simulink model "IEEE_9bus"  (R2018b)
settings: Solver=VariableStepAuto  StartTime=0.0  StopTime=10.0  FixedStep=0.0001  RelTol=1e-3
values from neighbouring files (symbols this model uses):
  R12 = 0.0180    (= 0.018)    [IEEE9BUSdata.m]
  R14 = 0.015    [IEEE9BUSdata.m]
  R23 = 0.018    [IEEE9BUSdata.m]
  R39 = 0.02    [IEEE9BUSdata.m]
  R45 = 0.013    [IEEE9BUSdata.m]
  R46 = 0.02    [IEEE9BUSdata.m]
  R57 = 0.014    [IEEE9BUSdata.m]
  R69 = 0.01    [IEEE9BUSdata.m]
  R78 = 0.032    [IEEE9BUSdata.m]
  R89 = 0.022    [IEEE9BUSdata.m]
  Xc12 = 0.0045    [IEEE9BUSdata.m]
  Xc14 = 0.0038    [IEEE9BUSdata.m]
  Xc23 = 0.00    (= 0)    [IEEE9BUSdata.m]
  Xc39 = 0.00    (= 0)    [IEEE9BUSdata.m]
  Xc45 = 0.003    [IEEE9BUSdata.m]
  Xc46 = 0.00    (= 0)    [IEEE9BUSdata.m]
  Xc57 = 0.003    [IEEE9BUSdata.m]
  Xc69 = 0.00    (= 0)    [IEEE9BUSdata.m]
  Xc78 = 0.00    (= 0)    [IEEE9BUSdata.m]
  Xc89 = 0.00    (= 0)    [IEEE9BUSdata.m]
  Xl12 = 0.054    [IEEE9BUSdata.m]
  Xl14 = 0.045    [IEEE9BUSdata.m]
  Xl23 = 0.056    [IEEE9BUSdata.m]
  Xl39 = 0.06    [IEEE9BUSdata.m]
  Xl45 = 0.036    [IEEE9BUSdata.m]
  Xl46 = 0.066    [IEEE9BUSdata.m]
  Xl57 = 0.036    [IEEE9BUSdata.m]
  Xl69 = 0.05    [IEEE9BUSdata.m]
  Xl78 = 0.076    [IEEE9BUSdata.m]
  Xl89 = 0.065    [IEEE9BUSdata.m]
libraries: powerlib x32
settings Model: Creator=033-18-0019  LastModifiedBy=033-18-0019

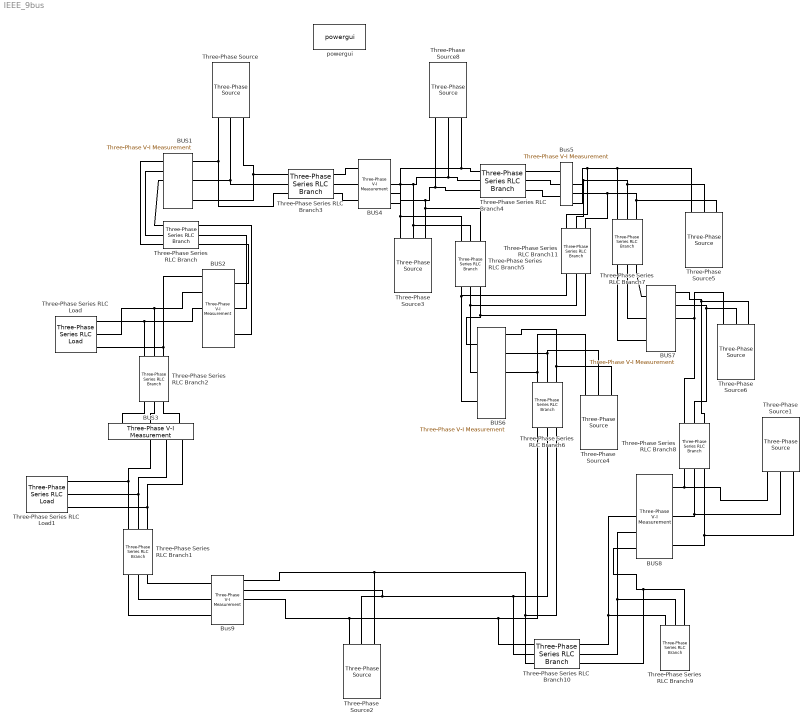
== system IEEE_9bus ==
  BUS1 : powerlib/Measurements/Three-Phase V-I Measurement  VoltageMeasurement=phase-to-ground  SetLabelV=off  LabelV=Vb1  Vpu=off  VpuLL=off  CurrentMeasurement=yes  SetLabelI=off  LabelI=Ib1  Ipu=off  Pbase=100e6  Vbase=500e3  OutputType=Complex  PhasorSimulation=off  PSBequivalent=0  mask(Three-Phase VI Measurement){}
      mask Display:
      | % This is a new mask on top of the base mask.
      | % Use "View base mask" link below to see the base mask.
      | disp('Bus1')
  BUS2 : powerlib/Measurements/Three-Phase V-I Measurement  VoltageMeasurement=phase-to-ground  SetLabelV=off  LabelV=Vabc  Vpu=off  VpuLL=off  CurrentMeasurement=yes  SetLabelI=off  LabelI=Iabc  Ipu=off  Pbase=100e6  Vbase=500e3  OutputType=Complex  PhasorSimulation=off  PSBequivalent=0  mask(Three-Phase VI Measurement){}
      mask Display:
      | % This is a new mask on top of the base mask.
      | % Use "View base mask" link below to see the base mask.
      | disp('Bus2')
  "BUS3 " : powerlib/Measurements/Three-Phase V-I Measurement  VoltageMeasurement=phase-to-ground  SetLabelV=off  LabelV=Vabc  Vpu=off  VpuLL=off  CurrentMeasurement=yes  SetLabelI=off  LabelI=Iabc  Ipu=off  Pbase=100e6  Vbase=500e3  OutputType=Complex  PhasorSimulation=off  PSBequivalent=0  mask(Three-Phase VI Measurement){}
      mask Display:
      | % This is a new mask on top of the base mask.
      | % Use "View base mask" link below to see the base mask.
      | disp('Bus3')
  BUS4 : powerlib/Measurements/Three-Phase V-I Measurement  VoltageMeasurement=phase-to-ground  SetLabelV=off  LabelV=Vb4  Vpu=on  VpuLL=off  CurrentMeasurement=yes  SetLabelI=off  LabelI=Ib4  Ipu=off  Pbase=100e6  Vbase=500e3  OutputType=Complex  PhasorSimulation=off  PSBequivalent=0
  BUS6 : powerlib/Measurements/Three-Phase V-I Measurement  VoltageMeasurement=phase-to-ground  SetLabelV=off  LabelV=Vb6  Vpu=on  VpuLL=off  CurrentMeasurement=yes  SetLabelI=off  LabelI=Ib6  Ipu=off  Pbase=100e6  Vbase=500e3  OutputType=Complex  PhasorSimulation=off  PSBequivalent=0
  BUS7 : powerlib/Measurements/Three-Phase V-I Measurement  VoltageMeasurement=phase-to-ground  SetLabelV=off  LabelV=Vb7  Vpu=on  VpuLL=off  CurrentMeasurement=yes  SetLabelI=off  LabelI=Ib7  Ipu=off  Pbase=100e6  Vbase=500e3  OutputType=Complex  PhasorSimulation=off  PSBequivalent=0
  BUS8 : powerlib/Measurements/Three-Phase V-I Measurement  VoltageMeasurement=phase-to-ground  SetLabelV=off  LabelV=Vb8  Vpu=off  VpuLL=off  CurrentMeasurement=yes  SetLabelI=off  LabelI=Ib8  Ipu=off  Pbase=100e6  Vbase=500e3  OutputType=Complex  PhasorSimulation=off  PSBequivalent=0
  Bus5 : powerlib/Measurements/Three-Phase V-I Measurement  VoltageMeasurement=phase-to-ground  SetLabelV=off  LabelV=V5  Vpu=on  VpuLL=off  CurrentMeasurement=yes  SetLabelI=off  LabelI=I5  Ipu=off  Pbase=100e6  Vbase=500e3  OutputType=Complex  PhasorSimulation=off  PSBequivalent=0
  Bus9 : powerlib/Measurements/Three-Phase V-I Measurement  VoltageMeasurement=phase-to-ground  SetLabelV=off  LabelV=Vb9  Vpu=on  VpuLL=off  CurrentMeasurement=yes  SetLabelI=off  LabelI=Ib9  Ipu=off  Pbase=100e6  Vbase=500e3  OutputType=Complex  PhasorSimulation=off  PSBequivalent=0
  Three-Phase Series RLC Branch : powerlib/Elements/Three-Phase Series RLC Branch  LConnTagsString=A|B|C  RConnTagsString=A|B|C  BranchType=RLC  Resistance=R12  Inductance=2*pi*50*Xl12  Capacitance=1/(2*pi*50*Xc12)  Measurements=None
  Three-Phase Series RLC Branch1 : powerlib/Elements/Three-Phase Series RLC Branch  LConnTagsString=A|B|C  RConnTagsString=A|B|C  BranchType=RLC  Resistance=R39  Inductance=2*pi*50*Xl39  Capacitance=1/(2*pi*50*Xc39)  Measurements=None
  Three-Phase Series RLC Branch10 : powerlib/Elements/Three-Phase Series RLC Branch  LConnTagsString=A|B|C  RConnTagsString=A|B|C  BranchType=RLC  Resistance=R89  Inductance=2*pi*50*Xl89  Capacitance=1/(2*pi*50*Xc89)  Measurements=None
  Three-Phase Series RLC Branch11 : powerlib/Elements/Three-Phase Series RLC Branch  LConnTagsString=A|B|C  RConnTagsString=A|B|C  BranchType=RLC  Resistance=R78  Inductance=2*pi*50*Xl78  Capacitance=1/(2*pi*50*Xc78)  Measurements=None
  Three-Phase Series RLC Branch2 : powerlib/Elements/Three-Phase Series RLC Branch  LConnTagsString=A|B|C  RConnTagsString=A|B|C  BranchType=RLC  Resistance=R23  Inductance=2*pi*50*Xl23  Capacitance=1/(2*pi*50*Xc23)  Measurements=None
  Three-Phase Series RLC Branch3 : powerlib/Elements/Three-Phase Series RLC Branch  LConnTagsString=A|B|C  RConnTagsString=A|B|C  BranchType=RLC  Resistance=R14  Inductance=2*pi*50*Xl14  Capacitance=1/(2*pi*50*Xc14)  Measurements=None
  Three-Phase Series RLC Branch4 : powerlib/Elements/Three-Phase Series RLC Branch  LConnTagsString=A|B|C  RConnTagsString=A|B|C  BranchType=RLC  Resistance=R45  Inductance=2*pi*50*Xl45  Capacitance=1/(2*pi*50*Xc45)  Measurements=None
  Three-Phase Series RLC Branch5 : powerlib/Elements/Three-Phase Series RLC Branch  LConnTagsString=A|B|C  RConnTagsString=A|B|C  BranchType=RLC  Resistance=R46  Inductance=2*pi*50*Xl46  Capacitance=1/(2*pi*50*Xc46)  Measurements=None
  Three-Phase Series RLC Branch6 : powerlib/Elements/Three-Phase Series RLC Branch  LConnTagsString=A|B|C  RConnTagsString=A|B|C  BranchType=RLC  Resistance=R69  Inductance=2*pi*50*Xl69  Capacitance=1/(2*pi*50*Xc69)  Measurements=None
  Three-Phase Series RLC Branch7 : powerlib/Elements/Three-Phase Series RLC Branch  LConnTagsString=A|B|C  RConnTagsString=A|B|C  BranchType=RLC  Resistance=R57  Inductance=2*pi*50*Xl57  Capacitance=1/(2*pi*50*Xc57)  Measurements=None
  Three-Phase Series RLC Branch8 : powerlib/Elements/Three-Phase Series RLC Branch  LConnTagsString=A|B|C  RConnTagsString=A|B|C  BranchType=RLC  Resistance=R78  Inductance=2*pi*50*Xl78  Capacitance=1/(2*pi*50*Xc78)  Measurements=None
  Three-Phase Series RLC Branch9 : powerlib/Elements/Three-Phase Series RLC Branch  LConnTagsString=A|B|C  RConnTagsString=A|B|C  BranchType=RLC  Resistance=R78  Inductance=2*pi*50*Xl78  Capacitance=1/(2*pi*50*Xc78)  Measurements=None
  Three-Phase Series RLC Load : powerlib/Elements/Three-Phase Series RLC Load  LConnTagsString=A|B|C  Configuration=Y (grounded)  NominalVoltage=1000  Vabc=[1e3 1e3 1e3]  Vabcp=[1e3 1e3 1e3]  NominalFrequency=60  UnbalancedPower=off  ActivePower=10e3  InductivePower=100  CapacitivePower=100  Pabc=[10e3 9e3 11e3]  QLabc=[100 90 110]  QCabc=[100 90 110]  Pabcp=[10e3 9e3 11e3]  QLabcp=[100 90 110]  QCabcp=[100 90 110]  Measurements=None  LoadType=constant Z
  Three-Phase Series RLC Load1 : powerlib/Elements/Three-Phase Series RLC Load  LConnTagsString=A|B|C  Configuration=Y (grounded)  NominalVoltage=1000  Vabc=[1e3 1e3 1e3]  Vabcp=[1e3 1e3 1e3]  NominalFrequency=60  UnbalancedPower=off  ActivePower=10e3  InductivePower=100  CapacitivePower=100  Pabc=[10e3 9e3 11e3]  QLabc=[100 90 110]  QCabc=[100 90 110]  Pabcp=[10e3 9e3 11e3]  QLabcp=[100 90 110]  QCabcp=[100 90 110]  Measurements=None  LoadType=constant Z
  Three-Phase Source : powerlib/Electrical Sources/Three-Phase Source  InternalConnection=Yg  VoltagePhases=off  Voltage=132e3  PhaseAngle=0  Voltage_phases=[25e3 25e3 25e3]/sqrt(3)  PhaseAngles_phases=[0 -120 +120]  Frequency=50  NonIdealSource=on  SpecifyImpedance=off  Resistance=0.8929  Inductance=0.05/(2*pi*50)  ShortCircuitLevel=100e6  BaseVoltage=132e3  XRratio=7  BusType=swing  Pref=10e3  Qref=0  Prefabc=[10e3, 10e3, 10e3]  Qrefabc=[0, 0, 0]  Qmin=-inf  Qmax=inf
  Three-Phase Source1 : powerlib/Electrical Sources/Three-Phase Source  InternalConnection=Yg  VoltagePhases=off  Voltage=132e3  PhaseAngle=0  Voltage_phases=[25e3 25e3 25e3]/sqrt(3)  PhaseAngles_phases=[0 -120 +120]  Frequency=50  NonIdealSource=on  SpecifyImpedance=off  Resistance=0.8929  Inductance=0.1/(2*pi*50)  ShortCircuitLevel=100e6  BaseVoltage=132e3  XRratio=7  BusType=swing  Pref=10e3  Qref=0  Prefabc=[10e3, 10e3, 10e3]  Qrefabc=[0, 0, 0]  Qmin=-inf  Qmax=inf
  Three-Phase Source{2..6} (5 alike) : powerlib/Electrical Sources/Three-Phase Source  InternalConnection=Yg  VoltagePhases=off  Voltage=25e3  PhaseAngle=0  Voltage_phases=[25e3 25e3 25e3]/sqrt(3)  PhaseAngles_phases=[0 -120 +120]  Frequency=60  NonIdealSource=on  SpecifyImpedance=off  Resistance=0.8929  Inductance=16.58e-3  ShortCircuitLevel=100e6  BaseVoltage=25e3  XRratio=7  BusType=swing  Pref=10e3  Qref=0  Prefabc=[10e3, 10e3, 10e3]  Qrefabc=[0, 0, 0]  Qmin=-inf  Qmax=inf
  Three-Phase Source8 : powerlib/Electrical Sources/Three-Phase Source  InternalConnection=Yg  VoltagePhases=off  Voltage=132e3  PhaseAngle=0  Voltage_phases=[25e3 25e3 25e3]/sqrt(3)  PhaseAngles_phases=[0 -120 +120]  Frequency=50  NonIdealSource=on  SpecifyImpedance=off  Resistance=0.8929  Inductance=0.08/(2*pi*50)  ShortCircuitLevel=100e6  BaseVoltage=132e3  XRratio=7  BusType=swing  Pref=10e3  Qref=0  Prefabc=[10e3, 10e3, 10e3]  Qrefabc=[0, 0, 0]  Qmin=-inf  Qmax=inf
  powergui : powerlib/powergui  Priority=1  SimulationMode=Discrete  SampleTime=50e-6  frequency=60  Iterations=50  frequencyindice=60  Pbase=100e6  ErrMax=1e-4  UnitsV=kV  UnitsW=MW  buscounter=0  FunctionMessages=off  echomessages=off  EnableUseOfTLC=off  CurrentSourceSwitches=off  DisableSnubberDevices=off  DisableRonSwitches=off  DisableVfSwitches=off  DisplayEquations=off  SolverType=Tustin/Backward Euler (TBE)  Interpol=off  ExternalGateDelay=off  methode=off  Ts=100  x0status=blocks  SPID=off  SwTol=0  HookPort=off  RestoreLinks=warning  ResistiveCurrentMeasurement=off  Frange=[0:2:500]  Ylog=off  Xlog=on  ShowGrid=off  save=off  variable=ZData  structure=0  ZoomFFT=off  StartTime=0.0  cycles=1  DisplayStyle=1  fundamental=60  FreqAxis=off  MaxFrequency=1000  frequencyindicesteady=1  RmsSteady=1  display=off
  connections:
  BUS4/LConn3 -- Three-Phase Series RLC Branch3/RConn3
  BUS4/LConn2 -- Three-Phase Series RLC Branch3/RConn2
  Three-Phase Source/RConn1 -- Three-Phase Series RLC Branch3/LConn1 -- BUS1/LConn1
  Three-Phase Series RLC Branch/RConn1 -- BUS2/LConn1
  Three-Phase Series RLC Branch/RConn2 -- BUS2/LConn2
  Three-Phase Series RLC Branch/RConn3 -- BUS2/LConn3
  Three-Phase Series RLC Branch/LConn1 -- BUS1/RConn1
  BUS1/RConn2 -- Three-Phase Series RLC Branch/LConn2
  BUS1/RConn3 -- Three-Phase Series RLC Branch/LConn3
  Three-Phase Series RLC Branch2/RConn1 -- "BUS3 "/LConn1
  "BUS3 "/LConn2 -- Three-Phase Series RLC Branch2/RConn2
  Three-Phase Series RLC Load/LConn3 -- BUS2/RConn3 -- Three-Phase Series RLC Branch2/LConn3
  "BUS3 "/RConn1 -- Three-Phase Series RLC Branch1/LConn1 -- Three-Phase Series RLC Load1/LConn1
  Three-Phase Series RLC Load1/LConn2 -- "BUS3 "/RConn2 -- Three-Phase Series RLC Branch1/LConn2
  "BUS3 "/RConn3 -- Three-Phase Series RLC Load1/LConn3 -- Three-Phase Series RLC Branch1/LConn3
  Three-Phase Series RLC Branch1/RConn1 -- Bus9/LConn1
  Three-Phase Series RLC Branch1/RConn2 -- Bus9/LConn2
  Three-Phase Series RLC Branch1/RConn3 -- Bus9/LConn3
  Three-Phase Series RLC Branch6/RConn1 -- Three-Phase Series RLC Branch10/RConn1 -- Bus9/RConn1 -- Three-Phase Source2/RConn1
  Three-Phase Series RLC Branch6/RConn2 -- Three-Phase Series RLC Branch10/RConn2 -- Three-Phase Source2/RConn2 -- Bus9/RConn2
  "BUS3 "/LConn3 -- Three-Phase Series RLC Branch2/RConn3
  Three-Phase Series RLC Load/LConn2 -- Three-Phase Series RLC Branch2/LConn2 -- BUS2/RConn2
  Three-Phase Series RLC Load/LConn1 -- Three-Phase Series RLC Branch2/LConn1 -- BUS2/RConn1
  BUS4/RConn1 -- Three-Phase Series RLC Branch4/LConn1 -- Three-Phase Source8/RConn1 -- Three-Phase Series RLC Branch5/LConn1 -- Three-Phase Source3/RConn1
  Three-Phase Source3/RConn2 -- Three-Phase Series RLC Branch5/LConn2 -- Three-Phase Series RLC Branch4/LConn2 -- Three-Phase Source8/RConn2 -- BUS4/RConn2
  Three-Phase Source3/RConn3 -- Three-Phase Series RLC Branch5/LConn3 -- Three-Phase Series RLC Branch4/LConn3 -- Three-Phase Source8/RConn3 -- BUS4/RConn3
  BUS4/LConn1 -- Three-Phase Series RLC Branch3/RConn1
  Three-Phase Source/RConn2 -- Three-Phase Series RLC Branch3/LConn2 -- BUS1/LConn2
  Three-Phase Series RLC Branch3/LConn3 -- BUS1/LConn3 -- Three-Phase Source/RConn3
  Three-Phase Series RLC Branch4/RConn1 -- Bus5/LConn1
  Three-Phase Series RLC Branch4/RConn2 -- Bus5/LConn2
  Three-Phase Series RLC Branch4/RConn3 -- Bus5/LConn3
  Three-Phase Series RLC Branch5/RConn1 -- BUS6/LConn1 -- Three-Phase Series RLC Branch11/RConn1
  Three-Phase Series RLC Branch5/RConn2 -- BUS6/LConn2 -- Three-Phase Series RLC Branch11/RConn2
  Three-Phase Series RLC Branch5/RConn3 -- Three-Phase Series RLC Branch11/RConn3 -- BUS6/LConn3
  BUS6/RConn1 -- Three-Phase Source4/RConn1 -- Three-Phase Series RLC Branch6/LConn1
  BUS6/RConn2 -- Three-Phase Source4/RConn2 -- Three-Phase Series RLC Branch6/LConn2
  BUS6/RConn3 -- Three-Phase Source4/RConn3 -- Three-Phase Series RLC Branch6/LConn3
  Three-Phase Series RLC Branch7/LConn1 -- Three-Phase Source5/RConn1 -- Three-Phase Series RLC Branch11/LConn1 -- Bus5/RConn1
  Three-Phase Series RLC Branch7/LConn2 -- Three-Phase Source5/RConn2 -- Three-Phase Series RLC Branch11/LConn2 -- Bus5/RConn2
  Three-Phase Series RLC Branch7/LConn3 -- Three-Phase Source5/RConn3 -- Bus5/RConn3 -- Three-Phase Series RLC Branch11/LConn3
  Three-Phase Series RLC Branch7/RConn1 -- BUS7/LConn1
  Three-Phase Series RLC Branch7/RConn2 -- BUS7/LConn2
  Three-Phase Series RLC Branch7/RConn3 -- BUS7/LConn3
  Three-Phase Source6/RConn1 -- Three-Phase Series RLC Branch8/LConn1 -- BUS7/RConn1
  Three-Phase Source6/RConn2 -- Three-Phase Series RLC Branch8/LConn2 -- BUS7/RConn2
  Three-Phase Source6/RConn3 -- Three-Phase Series RLC Branch8/LConn3 -- BUS7/RConn3
  Three-Phase Series RLC Branch8/RConn1 -- Three-Phase Source1/RConn1 -- BUS8/LConn1
  BUS8/LConn2 -- Three-Phase Source1/RConn2 -- Three-Phase Series RLC Branch8/RConn2
  BUS8/LConn3 -- Three-Phase Source1/RConn3 -- Three-Phase Series RLC Branch8/RConn3
  BUS8/RConn3 -- Three-Phase Series RLC Branch10/LConn3 -- Three-Phase Series RLC Branch9/LConn3
  Three-Phase Series RLC Branch9/LConn2 -- Three-Phase Series RLC Branch10/LConn2 -- BUS8/RConn2
  Three-Phase Series RLC Branch9/LConn1 -- BUS8/RConn1 -- Three-Phase Series RLC Branch10/LConn1
  Three-Phase Source2/RConn3 -- Three-Phase Series RLC Branch10/RConn3 -- Three-Phase Series RLC Branch6/RConn3 -- Bus9/RConn3
